simulink model "Lab5_Q1"  (R2021a)
settings: Solver=FixedStepDiscrete  StartTime=0.0  StopTime=10.0  FixedStep=1e-5  RelTol=1e-3
settings Model: Creator=student  LastModifiedBy=student

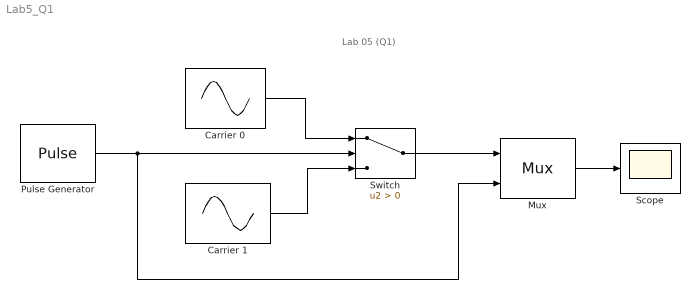
== system Lab5_Q1 ==
  note: Lab 05 (Q1)
  Carrier 0 : Sin  Frequency=40  SampleTime=0.01
  Carrier 1 : Sin  Frequency=10  SampleTime=0.01
  Mux : Mux  Inputs=2
  Pulse Generator : DiscretePulseGenerator  PulseType=Time based  PulseWidth=50
  Scope : Scope
  Switch : Switch  Criteria=u2 > Threshold
  wires:
  Pulse Generator/1 -> Mux/2, Switch/2
  Mux/1 -> Scope/1
  Switch/1 -> Mux/1
  Carrier 0/1 -> Switch/1
  Carrier 1/1 -> Switch/3
